simulink model "problem7app"  (R2020a)
settings: Solver=FixedStepAuto  StartTime=0.0  StopTime=10.0  FixedStep=0.2  RelTol=1e-3
settings Model: Creator=vijay  LastModifiedBy=vijay
settings DataIOCC: SaveOutput=off  SaveTime=off

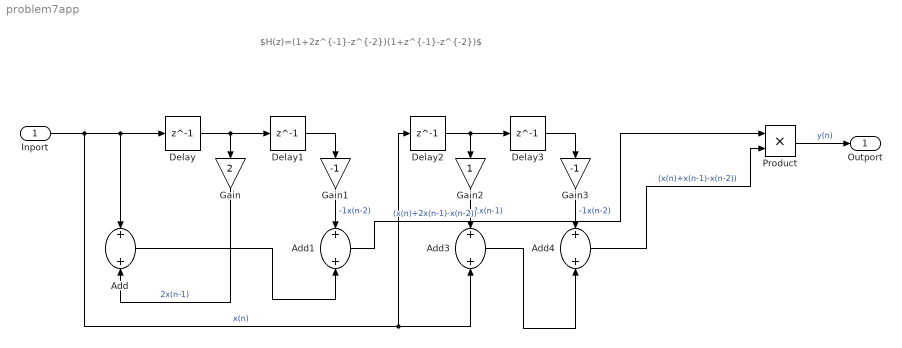
== system problem7app ==
  note: $H(z)=(1+2z^{-1}-z^{-2})(1+z^{-1}-z^{-2})$
  Inport : Inport  OutDataTypeStr=double  PortDimensions=1  SampleTime=[0.20000000000000001,0]
  Add{,1,3..4} (4 alike) : Sum
  Delay{,1..3} (4 alike) : Delay  DelayLength=1
  Gain : Gain  Gain=2
  Gain1 : Gain  Gain=-1
  Gain2 : Gain
  Gain3 : Gain  Gain=-1
  Product : Product
  Outport : Outport  OutDataTypeStr=double  PortDimensions=1  SampleTime=[0.20000000000000001,0]
  wires:
  Inport/1 -> Add/1, Delay/1, Add3/2, Delay2/1  "x(n)"
  Add3/1 -> Add4/2
  Delay3/1 -> Gain3/1
  Delay2/1 -> Gain2/1, Delay3/1
  Delay1/1 -> Gain1/1
  Add/1 -> Add1/2
  Delay/1 -> Gain/1, Delay1/1
  Gain1/1 -> Add1/1  "-1x(n-2)"
  Add4/1 -> Product/2  "(x(n)+x(n-1)-x(n-2))"
  Gain2/1 -> Add3/1  "1x(n-1)"
  Gain/1 -> Add/2  "2x(n-1)"
  Product/1 -> Outport/1  "y(n)"
  Gain3/1 -> Add4/1  "-1x(n-2)"
  Add1/1 -> Product/1  "(x(n)+2x(n-1)-x(n-2))"
